simulink model "PowerController"  (Simulink 7.6)
settings: Solver=ode45  StartTime=0.0  StopTime=10  FixedStep=Ts  RelTol=1e-3
undefined symbols (not defined in the file or in its folder): DiscIntNeverNeededParam, Hydride, Metal, Nickel
libraries: simulink x6, PECommon x4, powerlib x3, electricdrivelib x1
settings Model: Creator=Hu Xaiolei  LastModifiedBy=Hu Xaiolei
settings DebuggingCC: StrictBusMsg=Warning

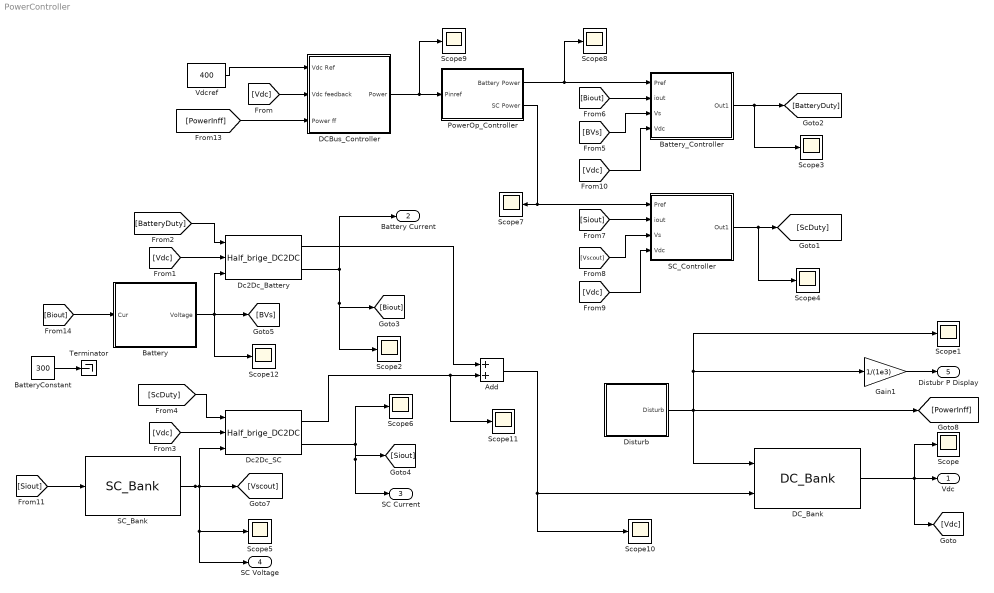
== system PowerController ==
  Add : Sum
  Battery : Subsystem  AncestorBlock=PECommon/Battery1  mask{Value=300}
      mask prompts: Value "Battery Normal Voltage"
      mask Display:
      | image(imread('D:\Work\NTU\matlab\PowerElectronics\pic\Battery_Service.jpg'))
      | port_label('input',1,'Current')
      | port_label('output',1,'Voltage')
  BatteryConstant : Constant  Value=300
  Battery_Controller : Subsystem  mask{Kp=0.0024999, Ki=0.0024999, imax=500, imin=-500}
  DCBus_Controller : Subsystem  mask{Kpdc=5905.8989, Kidc=1855.3929}
      mask prompts: Kpdc "Kp"; Kidc "Ki"
  DC_Bank : PECommon/DC_Bank  SystemSampleTime=-1  Cdc=0.47  Vdcinit=400
  Dc2Dc_Battery : PECommon/Half_brige_DC2DC  SystemSampleTime=-1  Ls=0.01  imax=500  imin=-500  Tsconv=0.0001
  Dc2Dc_SC : PECommon/Half_brige_DC2DC  SystemSampleTime=-1  Ls=0.001  imax=1200  imin=-1200  Tsconv=0.0001
  Disturb : Subsystem
      mask Display:
      | image(imread('D:\Work\NTU\matlab\PowerElectronics\pic\Load_Motor.jpg'))
      | port_label('output',1,'Disturb')
  Gain1 : Gain  Gain=1/(1e3)
  PowerOp_Controller : Subsystem  mask{Ts=0.001, DelayNum=1000, T=1, OmegaLP=62.8319}
      mask prompts: Ts "Sampling Rate"; DelayNum "Delay Num"; T "current Rising Time"; OmegaLP "Low Pass filter Cut off Freq"
  SC_Bank : PECommon/SC_Bank  SystemSampleTime=-1  CSC=4.4  Vscinit=254.951
  SC_Controller : Subsystem  mask{Kp=0.0024999, Ki=0.024999, imax=1200, imin=-1200}
  Scope{,1..12} (13 alike) : Scope
      Scope settings: SaveName=ScopeData2
      Scope1 settings: SaveName=ScopeData20
      Scope10 settings: SaveName=ScopeData12
      Scope11 settings: SaveName=ScopeData15
      Scope12 settings: SaveName=ScopeData13
      Scope2 settings: SaveName=ScopeData3
      Scope3 settings: SaveName=ScopeData6
      Scope4 settings: SaveName=ScopeData7
      Scope5 settings: SaveName=ScopeData4
      Scope6 settings: SaveName=ScopeData8
      Scope7 settings: SaveName=ScopeData9
      Scope8 settings: SaveName=ScopeData10
      Scope9 settings: SaveName=ScopeData11
  Terminator : Terminator
  Vdcref : Constant  Value=400
  Vdc : Outport
  Battery Current : Outport  Port=2
  SC Current : Outport  Port=3
  SC Voltage : Outport  Port=4
  Distubr P Display : Outport  Port=5
  wires:
  DC_Bank/1 -> Vdc/1, Scope/1, [Vdc]
  Vdcref/1 -> DCBus_Controller/1(Vdc Ref)
  [Vdc] -> DCBus_Controller/2(Vdc feedback)
  DCBus_Controller/1(Power) -> Scope9/1, PowerOp_Controller/1(Pinref)
  PowerOp_Controller/1(Battery Power) -> Battery_Controller/1(Pref), Scope8/1
  PowerOp_Controller/2(SC Power) -> Scope7/1, SC_Controller/1(Pref)
  Battery_Controller/1(Out1) -> [BatteryDuty], Scope3/1
  SC_Controller/1(Out1) -> [ScDuty], Scope4/1
  [Vdc] -> Dc2Dc_Battery/2
  [Vdc] -> Dc2Dc_SC/2
  [ScDuty] -> Dc2Dc_SC/1
  [BatteryDuty] -> Dc2Dc_Battery/1
  [Biout] -> Battery_Controller/2(iout)
  [BVs] -> Battery_Controller/3(Vs)
  [Vdc] -> SC_Controller/4(Vdc)
  [Vdc] -> Battery_Controller/4(Vdc)
  [Siout] -> SC_Controller/2(iout)
  [Vscout] -> SC_Controller/3(Vs)
  [Siout] -> SC_Bank/1
  Dc2Dc_SC/1 -> Add/2, Scope11/1
  Dc2Dc_Battery/1 -> Add/1
  Dc2Dc_Battery/2 -> [Biout], Scope2/1, Battery Current/1
  Dc2Dc_SC/2 -> Scope6/1, SC Current/1, [Siout]
  Disturb/1(Disturb) -> [PowerInff], Scope1/1, Gain1/1, DC_Bank/1
  [PowerInff] -> DCBus_Controller/3(Power ff)
  Gain1/1 -> Distubr P Display/1
  Battery/1(Voltage) -> Dc2Dc_Battery/3, [BVs], Scope12/1
  [Biout] -> Battery/1(Cur)
  BatteryConstant/1 -> Terminator/1
  SC_Bank/1 -> [Vscout], Dc2Dc_SC/3, Scope5/1, SC Voltage/1
  Add/1 -> Scope10/1, DC_Bank/2

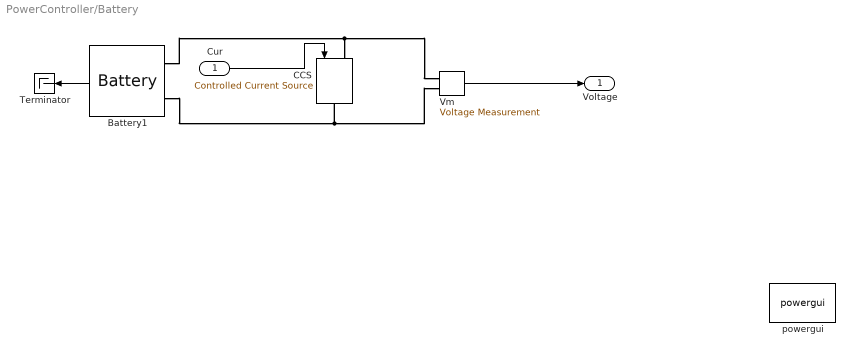
== system PowerController/Battery ==
  Cur : Inport
  Battery1 : electricdrivelib/Extra Sources/Battery  DialogController=POWERSYS.PowerSysDialog  SystemSampleTime=-1  BatType=Nickel-Metal-Hydride  ShowDetailedParameters=off  NomV=Value  NomQ=1000  SOC=70  PresetModel=on  MaxQ=1076.9231  FullV=353.3898  Dis_rate=200  R=0.003  Normal_OP=961.5385  expZone="[325.4237           200]"  Dis_Char=off  current=[1.5 3]  Units=Ampere-hour  Batt_Tr=30
  CCS : powerlib/Electrical Sources/Controlled Current Source  DialogController=POWERSYS.PowerSysDialog  SystemSampleTime=-1  Initialize=off  Source_Type=DC  Amplitude=0  Phase=0  Frequency=0  Measurements=None
  Terminator : Terminator
  Vm : powerlib/Measurements/Voltage Measurement  DialogController=POWERSYS.PowerSysDialog  SystemSampleTime=-1  PhasorSimulation=off  OutputType=Complex  PSBequivalent=0
  powergui : powerlib/powergui  Priority=1  SystemSampleTime=-1  SimulationMode=Continuous  SampleTime=50e-6  frequency=60  SPID=off  DisableSnubberDevices=off  DisableRonSwitches=off  DisableVfSwitches=off  SwTol=0  Interpol=off  frequencyindice=0  echomessages=off  HookPort=off  DisplayEquations=off  FunctionMessages=off  EnableUseOfTLC=off  x0status=blocks  RestoreLinks=warning  ResistiveCurrentMeasurement=off  Ylog=off  Xlog=on  ShowGrid=off  save=off  variable=ZData  ZoomFFT=off  StartTime=0.0  cycles=1  DisplayStyle=1  FreqAxis=off  MaxFrequency=1000  frequencyindicesteady=1  display=off  methode=off
  Voltage : Outport
  wires:
  Battery1/1 -> Terminator/1
  Vm/1 -> Voltage/1
  Cur/1 -> CCS/1
  connections:
  Battery1/LConn1 -- CCS/LConn1 -- Vm/LConn1
  Battery1/LConn2 -- CCS/RConn1 -- Vm/LConn2

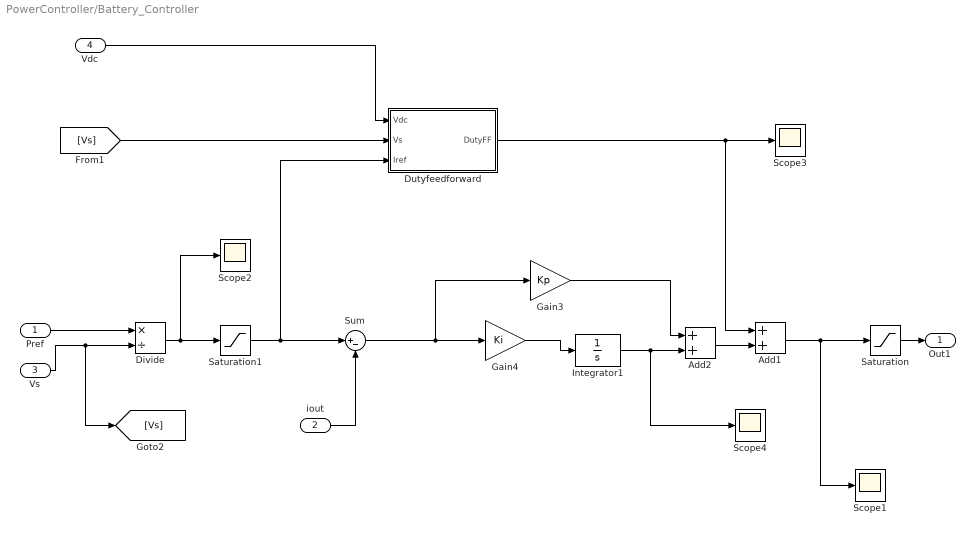
== system PowerController/Battery_Controller ==
  Pref : Inport
  iout : Inport  Port=2
  Vs : Inport  Port=3
  Vdc : Inport  Port=4
  Add1 : Sum
  Add2 : Sum
  Divide : Product  Inputs=*/
  Dutyfeedforward : Subsystem
  Gain3 : Gain  Gain=Kp
  Gain4 : Gain  Gain=Ki
  Integrator1 : Integrator
  Saturation : Saturate  UpperLimit=1  LowerLimit=-1
  Saturation1 : Saturate  UpperLimit=imax  LowerLimit=imin
  Scope{1..4} (4 alike) : Scope
      Scope1 settings: SaveName=ScopeData6
      Scope2 settings: SaveName=ScopeData5
      Scope3 settings: SaveName=ScopeData7
      Scope4 settings: SaveName=ScopeData22
  Sum : Sum  Inputs=|+-
  Out1 : Outport
  wires:
  iout/1 -> Sum/2
  Divide/1 -> Scope2/1, Saturation1/1
  Pref/1 -> Divide/1
  Saturation/1 -> Out1/1
  Vs/1 -> Divide/2, [Vs]
  Dutyfeedforward/1(DutyFF) -> Add1/1, Scope3/1
  Vdc/1 -> Dutyfeedforward/1(Vdc)
  [Vs] -> Dutyfeedforward/2(Vs)
  Add1/1 -> Saturation/1, Scope1/1
  Sum/1 -> Gain4/1, Gain3/1
  Gain4/1 -> Integrator1/1
  Gain3/1 -> Add2/1
  Integrator1/1 -> Add2/2, Scope4/1
  Add2/1 -> Add1/2
  Saturation1/1 -> Sum/1, Dutyfeedforward/3(Iref)

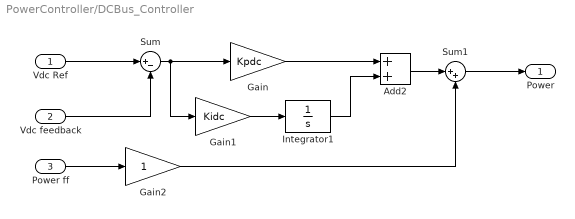
== system PowerController/DCBus_Controller ==
  Vdc Ref : Inport
  Vdc feedback : Inport  Port=2
  Power ff : Inport  Port=3
  Add2 : Sum
  Gain : Gain  Gain=Kpdc
  Gain1 : Gain  Gain=Kidc
  Gain2 : Gain
  Integrator1 : Integrator
  Sum : Sum  Inputs=|+-
  Sum1 : Sum  Inputs=|++
  Power : Outport
  wires:
  Gain/1 -> Add2/1
  Sum/1 -> Gain/1, Gain1/1
  Vdc Ref/1 -> Sum/1
  Vdc feedback/1 -> Sum/2
  Gain1/1 -> Integrator1/1
  Integrator1/1 -> Add2/2
  Sum1/1 -> Power/1
  Power ff/1 -> Gain2/1
  Add2/1 -> Sum1/1
  Gain2/1 -> Sum1/2

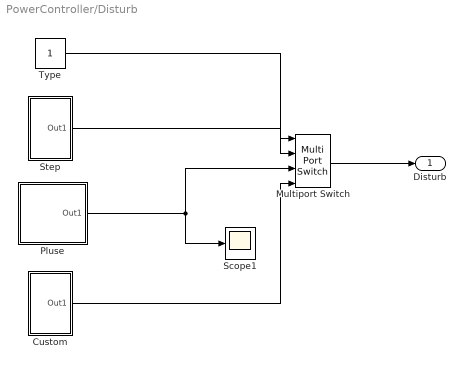
== system PowerController/Disturb ==
  Custom : Subsystem  mask{Value=[100,-100,0,50,-50,0], TsCustom=5}
      mask prompts: Value "Value kw"; TsCustom "Step Time"
  Multiport Switch : MultiPortSwitch  zeroidx=off
  Pluse : Subsystem  mask{MaxP=100, MinP=-100, PluseTs=0.1}
      mask prompts: MaxP "Max Power kw"; MinP "Min Power kw"; PluseTs "Duration"
  Scope1 : Scope
  Step : Subsystem  mask{InitP=0, FinalP=100, StepT=0}
      mask prompts: InitP "Initial Power kw"; FinalP "Final Power kw"; StepT "Step Time kw"
  Type : Constant
  Disturb : Outport
  wires:
  Custom/1(Out1) -> Multiport Switch/4
  Pluse/1(Out1) -> Scope1/1, Multiport Switch/3
  Step/1(Out1) -> Multiport Switch/2
  Multiport Switch/1 -> Disturb/1
  Type/1 -> Multiport Switch/1

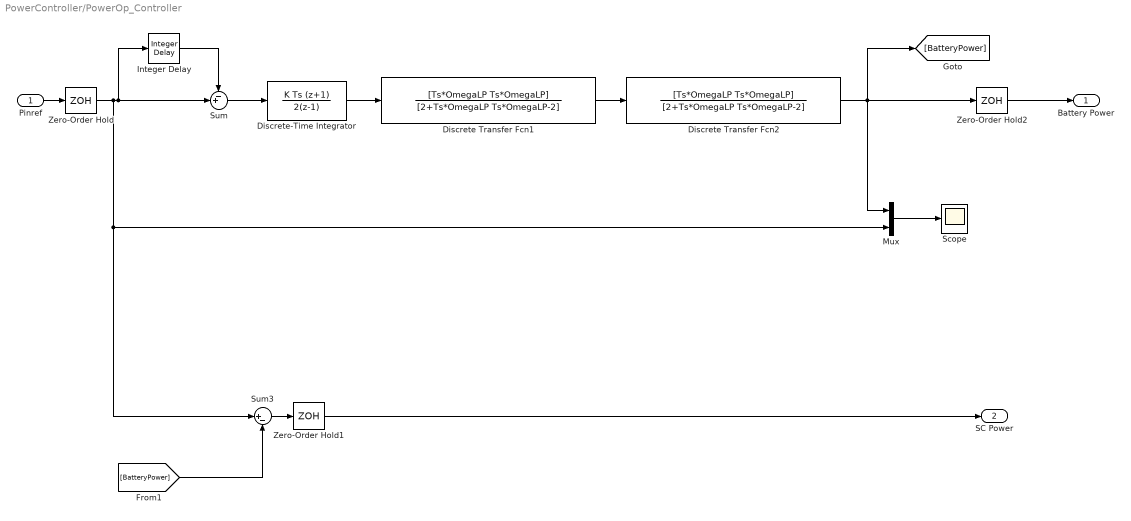
== system PowerController/PowerOp_Controller ==
  Pinref : Inport
  Discrete Transfer Fcn1 : DiscreteTransferFcn  Numerator=[Ts*OmegaLP Ts*OmegaLP]  Denominator=[2+Ts*OmegaLP Ts*OmegaLP-2]  SampleTime=Ts
  Discrete Transfer Fcn2 : DiscreteTransferFcn  Numerator=[Ts*OmegaLP Ts*OmegaLP]  Denominator=[2+Ts*OmegaLP Ts*OmegaLP-2]  SampleTime=Ts
  Discrete-Time Integrator : DiscreteIntegrator  IntegratorMethod=Integration: Trapezoidal  gainval=1/T  SampleTime=Ts  ICPrevOutput=DiscIntNeverNeededParam  ICPrevScaledInput=DiscIntNeverNeededParam
  Integer Delay : simulink/Discrete/Integer Delay  NumDelays=DelayNum  InputProcessing=Inherited  vinit=0.0  samptime=Ts
  Mux : Mux  Inputs=2
  Scope : Scope
      settings: TimeRange=2.393038433647571  YMin=0  YMax=0.5
  Sum : Sum  Inputs=-+|
  Sum3 : Sum  Inputs=|+-
  Zero-Order Hold : ZeroOrderHold  SampleTime=Ts
  Zero-Order Hold1 : ZeroOrderHold  SampleTime=Ts
  Zero-Order Hold2 : ZeroOrderHold  SampleTime=Ts
  Battery Power : Outport
  SC Power : Outport  Port=2
  wires:
  Mux/1 -> Scope/1
  [BatteryPower] -> Sum3/2
  Zero-Order Hold/1 -> Sum3/1, Mux/2, Sum/2, Integer Delay/1
  Discrete-Time Integrator/1 -> Discrete Transfer Fcn1/1
  Sum/1 -> Discrete-Time Integrator/1
  Integer Delay/1 -> Sum/1
  Pinref/1 -> Zero-Order Hold/1
  Sum3/1 -> Zero-Order Hold1/1
  Zero-Order Hold2/1 -> Battery Power/1
  Zero-Order Hold1/1 -> SC Power/1
  Discrete Transfer Fcn2/1 -> Mux/1, [BatteryPower], Zero-Order Hold2/1
  Discrete Transfer Fcn1/1 -> Discrete Transfer Fcn2/1

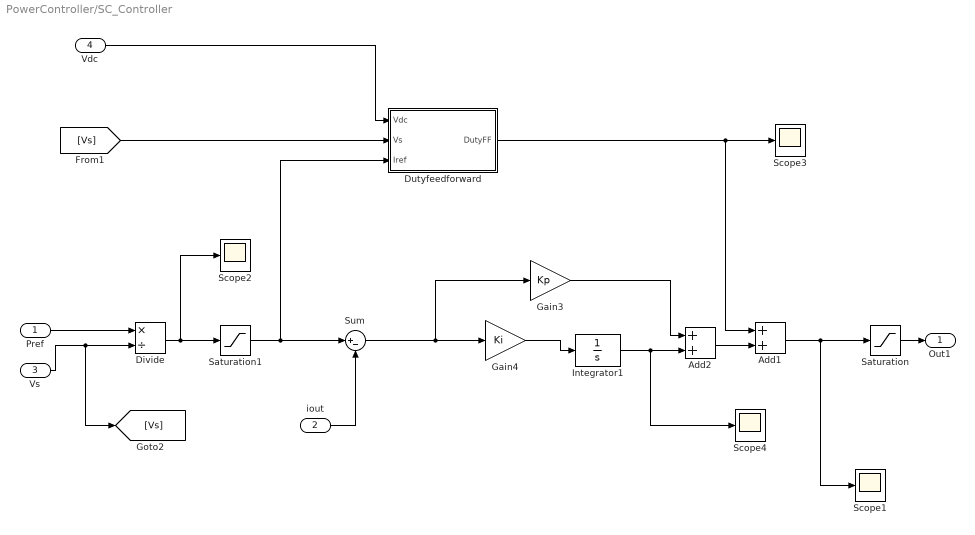
== system PowerController/SC_Controller ==
  Pref : Inport
  iout : Inport  Port=2
  Vs : Inport  Port=3
  Vdc : Inport  Port=4
  Add1 : Sum
  Add2 : Sum
  Divide : Product  Inputs=*/
  Dutyfeedforward : Subsystem
  Gain3 : Gain  Gain=Kp
  Gain4 : Gain  Gain=Ki
  Integrator1 : Integrator
  Saturation : Saturate  UpperLimit=1  LowerLimit=-1
  Saturation1 : Saturate  UpperLimit=imax  LowerLimit=imin
  Scope{1..4} (4 alike) : Scope
      Scope1 settings: SaveName=ScopeData6
      Scope2 settings: SaveName=ScopeData5
      Scope3 settings: SaveName=ScopeData7
      Scope4 settings: SaveName=ScopeData22
  Sum : Sum  Inputs=|+-
  Out1 : Outport
  wires:
  Saturation1/1 -> Dutyfeedforward/3(Iref), Sum/1
  Add2/1 -> Add1/2
  Integrator1/1 -> Scope4/1, Add2/2
  Gain3/1 -> Add2/1
  Gain4/1 -> Integrator1/1
  Sum/1 -> Gain3/1, Gain4/1
  Add1/1 -> Scope1/1, Saturation/1
  [Vs] -> Dutyfeedforward/2(Vs)
  Vdc/1 -> Dutyfeedforward/1(Vdc)
  Dutyfeedforward/1(DutyFF) -> Scope3/1, Add1/1
  Vs/1 -> [Vs], Divide/2
  Saturation/1 -> Out1/1
  Pref/1 -> Divide/1
  Divide/1 -> Saturation1/1, Scope2/1
  iout/1 -> Sum/2

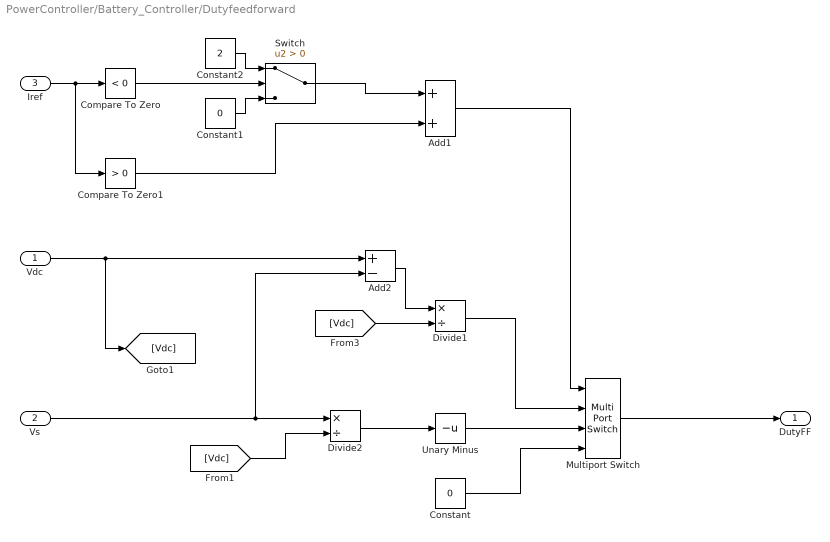
== system PowerController/Battery_Controller/Dutyfeedforward ==
  Vdc : Inport
  Vs : Inport  Port=2
  Iref : Inport  Port=3
  Add1 : Sum
  Add2 : Sum  Inputs=+-
  Compare To Zero : simulink/Logic and Bit Operations/Compare To Zero  SystemSampleTime=-1  relop=<  LogicOutDataTypeMode=boolean
  Compare To Zero1 : simulink/Logic and Bit Operations/Compare To Zero  SystemSampleTime=-1  relop=>  LogicOutDataTypeMode=boolean
  Constant : Constant  Value=0
  Constant1 : Constant  Value=0
  Constant2 : Constant  Value=2
  Divide1 : Product  Inputs=*/
  Divide2 : Product  Inputs=*/
  Multiport Switch : MultiPortSwitch  DiagnosticForDefault=None  zeroidx=off
  Switch : Switch  Criteria=u2 > Threshold
  Unary Minus : UnaryMinus
  DutyFF : Outport
  wires:
  Vdc/1 -> Add2/1, [Vdc]
  Add2/1 -> Divide1/1
  [Vdc] -> Divide1/2
  Divide2/1 -> Unary Minus/1
  Divide1/1 -> Multiport Switch/2
  Unary Minus/1 -> Multiport Switch/3
  Constant/1 -> Multiport Switch/4
  Multiport Switch/1 -> DutyFF/1
  Iref/1 -> Compare To Zero/1, Compare To Zero1/1
  Compare To Zero/1 -> Switch/2
  Constant2/1 -> Switch/1
  Constant1/1 -> Switch/3
  Compare To Zero1/1 -> Add1/2
  Switch/1 -> Add1/1
  Add1/1 -> Multiport Switch/1
  Vs/1 -> Divide2/1, Add2/2
  [Vdc] -> Divide2/2

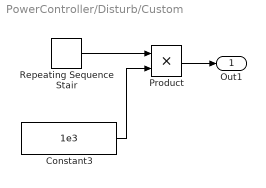
== system PowerController/Disturb/Custom ==
  Constant3 : Constant  Value=1e3
  Product : Product  RndMeth=Zero
  Repeating Sequence Stair : simulink/Sources/Repeating Sequence Stair  SystemSampleTime=-1  OutValues=Value.'  tsamp=TsCustom  OutMin=[]  OutMax=[]  OutDataTypeStr=double  OutputDataTypeScalingMode=double  OutDataType=fixdt(0,8)  ConRadixGroup=Best Precision: Vector-wise  OutScaling=2^-12
  Out1 : Outport
  wires:
  Constant3/1 -> Product/2
  Product/1 -> Out1/1
  Repeating Sequence Stair/1 -> Product/1

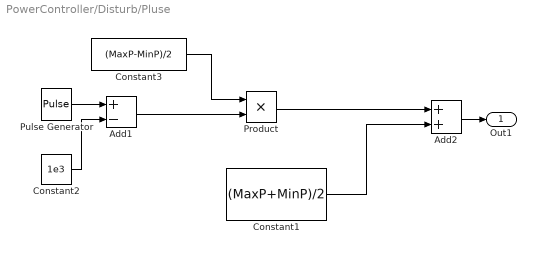
== system PowerController/Disturb/Pluse ==
  Add1 : Sum  Inputs=+-
  Add2 : Sum
  Constant1 : Constant  Value=(MaxP+MinP)/2
  Constant2 : Constant  Value=1e3
  Constant3 : Constant  Value=(MaxP-MinP)/2
  Product : Product  RndMeth=Zero
  Pulse Generator : DiscretePulseGenerator  PulseType=Time based  Amplitude=2e3  Period=PluseTs  PulseWidth=50
  Out1 : Outport
  wires:
  Constant1/1 -> Add2/2
  Add2/1 -> Out1/1
  Product/1 -> Add2/1
  Constant3/1 -> Product/1
  Add1/1 -> Product/2
  Constant2/1 -> Add1/2
  Pulse Generator/1 -> Add1/1

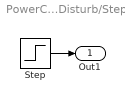
== system PowerController/Disturb/Step ==
  Step : Step  Time=StepT  Before=InitP*1e3  After=FinalP*1e3  SampleTime=0
  Out1 : Outport
  wires:
  Step/1 -> Out1/1

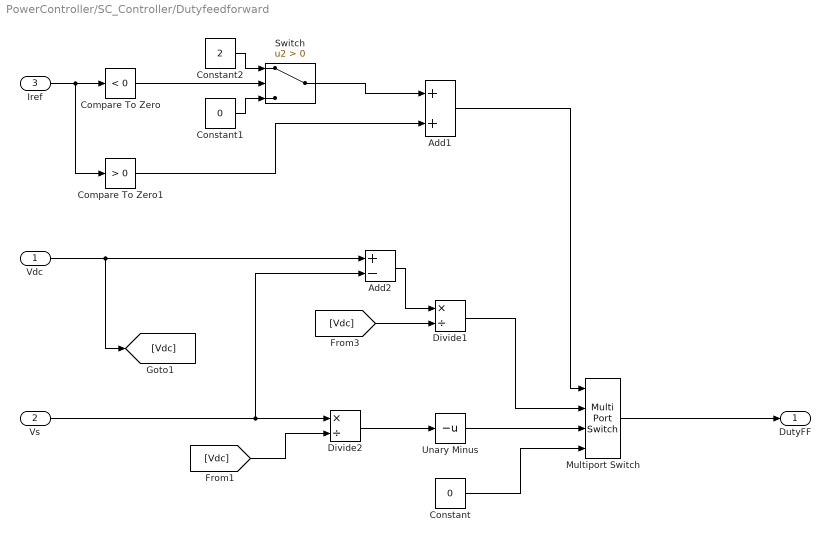
== system PowerController/SC_Controller/Dutyfeedforward ==
  Vdc : Inport
  Vs : Inport  Port=2
  Iref : Inport  Port=3
  Add1 : Sum
  Add2 : Sum  Inputs=+-
  Compare To Zero : simulink/Logic and Bit Operations/Compare To Zero  SystemSampleTime=-1  relop=<  LogicOutDataTypeMode=boolean
  Compare To Zero1 : simulink/Logic and Bit Operations/Compare To Zero  SystemSampleTime=-1  relop=>  LogicOutDataTypeMode=boolean
  Constant : Constant  Value=0
  Constant1 : Constant  Value=0
  Constant2 : Constant  Value=2
  Divide1 : Product  Inputs=*/
  Divide2 : Product  Inputs=*/
  Multiport Switch : MultiPortSwitch  DiagnosticForDefault=None  zeroidx=off
  Switch : Switch  Criteria=u2 > Threshold
  Unary Minus : UnaryMinus
  DutyFF : Outport
  wires:
  [Vdc] -> Divide2/2
  Vs/1 -> Add2/2, Divide2/1
  Add1/1 -> Multiport Switch/1
  Switch/1 -> Add1/1
  Compare To Zero1/1 -> Add1/2
  Constant1/1 -> Switch/3
  Constant2/1 -> Switch/1
  Compare To Zero/1 -> Switch/2
  Iref/1 -> Compare To Zero1/1, Compare To Zero/1
  Multiport Switch/1 -> DutyFF/1
  Constant/1 -> Multiport Switch/4
  Unary Minus/1 -> Multiport Switch/3
  Divide1/1 -> Multiport Switch/2
  Divide2/1 -> Unary Minus/1
  [Vdc] -> Divide1/2
  Add2/1 -> Divide1/1
  Vdc/1 -> [Vdc], Add2/1
